simulink library "StateEstimation_lib"  (R2016b)
settings: Solver=VariableStepAuto  StartTime=0.0  StopTime=10.0  RelTol=1e-3
values from neighbouring files (symbols this model uses):
  accel_bias_init = zeros(3,1)    [Copy_of_StateEstimator_RIEKF.m]    (also in Quaternion_EKF.m; RightInvariant_EKF.m; StateEstimator_EKF.m; StateEstimator_RIEKF.m)
  accel_bias_noise_std = 0.1*ones(3,1)    [Copy_of_StateEstimator_RIEKF.m]    (also in Quaternion_EKF.m; RightInvariant_EKF.m; StateEstimator_EKF.m; StateEstimator_RIEKF.m)
  accel_noise_std = 0.1*ones(3,1)    [Copy_of_StateEstimator_RIEKF.m]    (also in Quaternion_EKF.m; RightInvariant_EKF.m; StateEstimator_EKF.m; StateEstimator_RIEKF.m)
  gyro_bias_init = zeros(3,1)    [Copy_of_StateEstimator_RIEKF.m]    (also in Quaternion_EKF.m; RightInvariant_EKF.m; StateEstimator_EKF.m; StateEstimator_RIEKF.m)
  gyro_bias_noise_std = 0.1*ones(3,1)    [Copy_of_StateEstimator_RIEKF.m]    (also in Quaternion_EKF.m; RightInvariant_EKF.m; StateEstimator_EKF.m; StateEstimator_RIEKF.m)
  gyro_noise_std = 0.1*ones(3,1)    [Copy_of_StateEstimator_RIEKF.m]    (also in Quaternion_EKF.m; RightInvariant_EKF.m; StateEstimator_EKF.m; StateEstimator_RIEKF.m)
undefined symbols (not defined in the file or in its folder): cassieParameters, CassieParameters, EKF_SampleTime, q_init, v_init
libraries: xpcutilitieslib x41, xpcrtudplib x41, dspfdesign x10, simulink x6, slrtlib x5
(part 1 of 4)
settings Model: Creator=Ross Hartley  LastModifiedBy=Ross Hartley

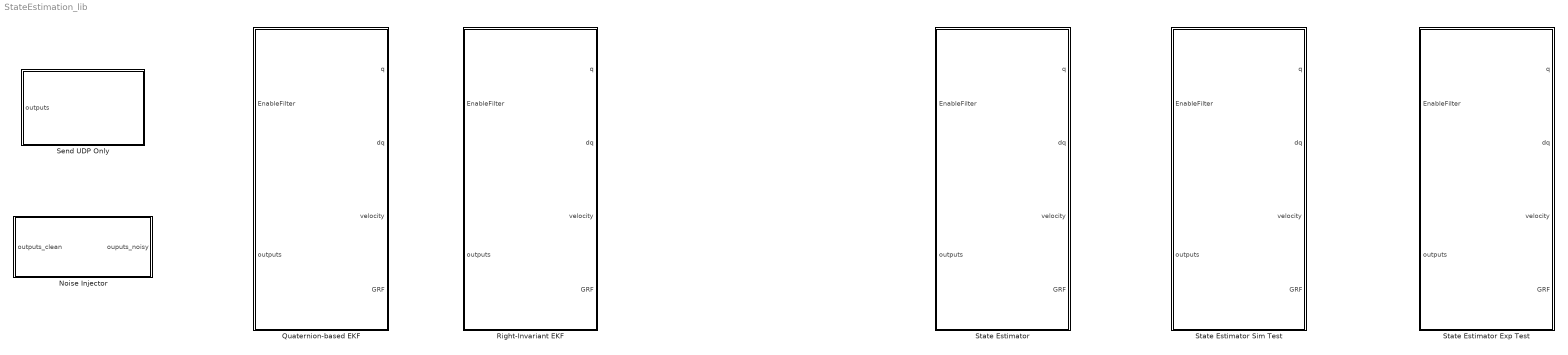
== system StateEstimation_lib ==
  Noise Injector : Subsystem
  Quaternion-based EKF : Subsystem
  Right-Invariant EKF : Subsystem
  Send UDP Only : Subsystem
  State Estimator : Subsystem
  State Estimator Exp Test : Subsystem
  State Estimator Sim Test : Subsystem

== system StateEstimation_lib/Noise Injector ==
  outputs_clean : Inport
  Bus Creator : BusCreator  Inputs=13  OutDataTypeStr=Bus: cassieOutputsBus
  Bus Selector1 : BusSelector  OutputSignals=vectorNavOrientation,vectorNavAngularVelocity,vectorNavLinearAcceleration,vectorNavMagneticField,vectorNavPressure,vectorNavTemperature,motorPosition,motorVelocity,jointPosition,jointVelocity,radio,stateOfCharge,status
  Inject Angular Velocity Noise : Subsystem
  Inject Linear Acceleration Noise : Subsystem
  ouputs_noisy : Outport
  wires:
  Inject Linear Acceleration Noise/1(a_noisy) -> Bus Creator/3  "vectorNavLinearAcceleration"
  Inject Angular Velocity Noise/1(w_noisy) -> Bus Creator/2  "vectorNavAngularVelocity"
  Bus Selector1/2 -> Inject Angular Velocity Noise/1(w_clean)  "<vectorNavAngularVelocity>"
  Bus Creator/1 -> ouputs_noisy/1
  outputs_clean/1 -> Bus Selector1/1
  Bus Selector1/11 -> Bus Creator/11  "<radio>"
  Bus Selector1/12 -> Bus Creator/12  "<stateOfCharge>"
  Bus Selector1/9 -> Bus Creator/9  "<jointPosition>"
  Bus Selector1/13 -> Bus Creator/13  "<status>"
  Bus Selector1/10 -> Bus Creator/10  "<jointVelocity>"
  Bus Selector1/8 -> Bus Creator/8  "<motorVelocity>"
  Bus Selector1/3 -> Inject Linear Acceleration Noise/1(a_clean)  "<vectorNavLinearAcceleration>"
  Bus Selector1/4 -> Bus Creator/4  "<vectorNavMagneticField>"
  Bus Selector1/7 -> Bus Creator/7  "<motorPosition>"
  Bus Selector1/5 -> Bus Creator/5  "<vectorNavPressure>"
  Bus Selector1/6 -> Bus Creator/6  "<vectorNavTemperature>"
  Bus Selector1/1 -> Bus Creator/1  "<vectorNavOrientation>"

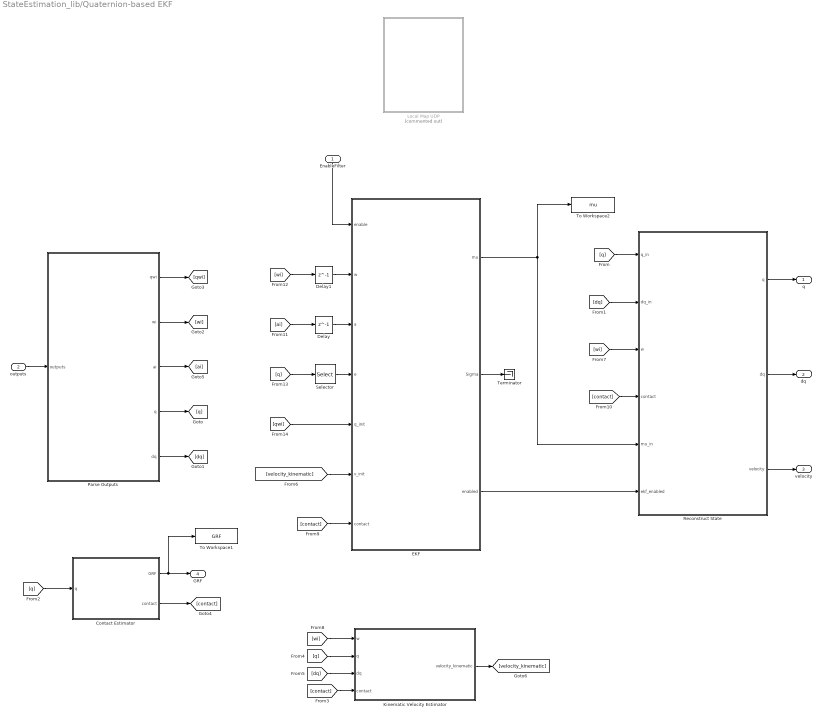
== system StateEstimation_lib/Quaternion-based EKF ==
  EnableFilter : Inport
  outputs : Inport  Port=2
  Contact Estimator : Subsystem
  Delay : Delay  DelayLength=1  InitialCondition=0
  Delay1 : Delay  DelayLength=1  InitialCondition=0
  EKF : Subsystem
  Kinematic Velocity Estimator : Subsystem
  Local Map UDP : Subsystem  Commented=on
  Parse Outputs : Subsystem
  Reconstruct State : Subsystem
  Selector : Selector  InputPortWidth=20  IndexOptions=Index vector (dialog)  Indices=[7:20]  OutputSizes=1
  Terminator : Terminator
  To Workspace1 : ToWorkspace  VariableName=GRF  SaveFormat=Timeseries  SampleTime=-1
  To Workspace2 : ToWorkspace  VariableName=mu  SaveFormat=Timeseries  SampleTime=-1
  q : Outport
  dq : Outport  Port=2
  velocity : Outport  Port=3
  GRF : Outport  Port=4
  wires:
  EKF/2(Sigma) -> Terminator/1
  EnableFilter/1 -> EKF/1(enable)
  [contact] -> EKF/7(contact)
  [ai] -> Delay/1
  [wi] -> Delay1/1
  [q] -> Selector/1
  outputs/1 -> Parse Outputs/1(outputs)
  Parse Outputs/3(ai) -> [ai]
  Parse Outputs/2(wi) -> [wi]
  Parse Outputs/4(q) -> [q]
  Parse Outputs/5(dq) -> [dq]
  Parse Outputs/1(qwi) -> [qwi]
  [q] -> Reconstruct State/1(q_in)
  [dq] -> Reconstruct State/2(dq_in)
  EKF/3(enabled) -> Reconstruct State/6(ekf_enabled)
  Reconstruct State/1(q) -> q/1
  Reconstruct State/2(dq) -> dq/1
  Reconstruct State/3(velocity) -> velocity/1
  Delay1/1 -> EKF/2(w)
  [wi] -> Reconstruct State/3(w)
  [contact] -> Reconstruct State/4(contact)
  [q] -> Contact Estimator/1(q)
  Contact Estimator/1(GRF) -> To Workspace1/1, GRF/1
  Contact Estimator/2(contact) -> [contact]
  EKF/1(mu) -> To Workspace2/1, Reconstruct State/5(mu_in)
  [wi] -> Kinematic Velocity Estimator/1(w)
  [q] -> Kinematic Velocity Estimator/2(q)
  [dq] -> Kinematic Velocity Estimator/3(dq)
  [contact] -> Kinematic Velocity Estimator/4(contact)
  Kinematic Velocity Estimator/1(velocity_kinematic) -> [velocity_kinematic]
  Delay/1 -> EKF/3(a)
  Selector/1 -> EKF/4(e)
  [qwi] -> EKF/5(q_init)
  [velocity_kinematic] -> EKF/6(v_init)

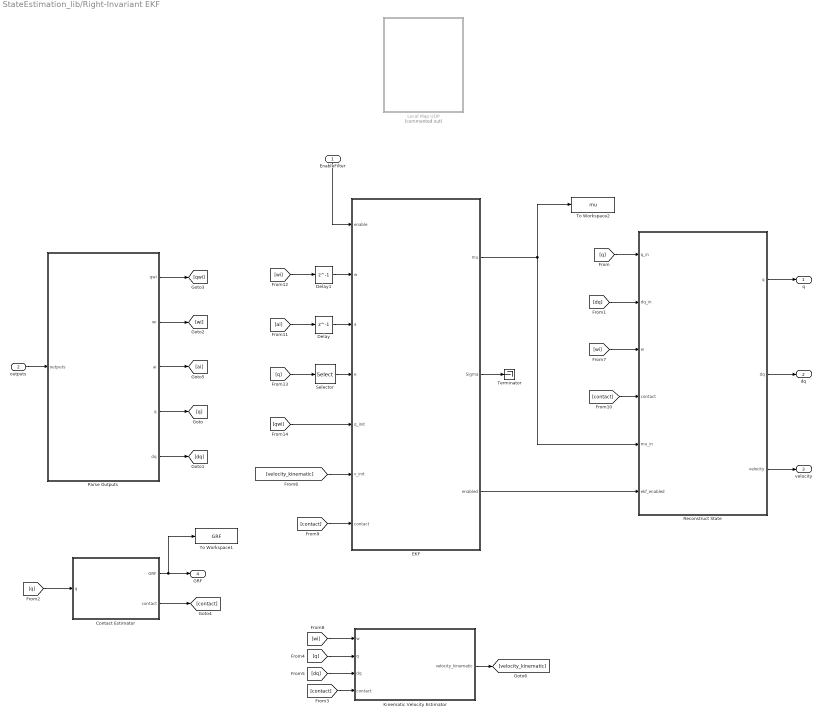
== system StateEstimation_lib/Right-Invariant EKF ==
  EnableFilter : Inport
  outputs : Inport  Port=2
  Contact Estimator : Subsystem
  Delay : Delay  DelayLength=1  InitialCondition=0
  Delay1 : Delay  DelayLength=1  InitialCondition=0
  EKF : Subsystem
  Kinematic Velocity Estimator : Subsystem
  Local Map UDP : Subsystem  Commented=on
  Parse Outputs : Subsystem
  Reconstruct State : Subsystem
  Selector : Selector  InputPortWidth=20  IndexOptions=Index vector (dialog)  Indices=[7:20]  OutputSizes=1
  Terminator : Terminator
  To Workspace1 : ToWorkspace  VariableName=GRF  SaveFormat=Timeseries  SampleTime=-1
  To Workspace2 : ToWorkspace  VariableName=mu  SaveFormat=Timeseries  SampleTime=-1
  q : Outport
  dq : Outport  Port=2
  velocity : Outport  Port=3
  GRF : Outport  Port=4
  wires:
  EKF/2(Sigma) -> Terminator/1
  EnableFilter/1 -> EKF/1(enable)
  [contact] -> EKF/7(contact)
  [ai] -> Delay/1
  [wi] -> Delay1/1
  [q] -> Selector/1
  outputs/1 -> Parse Outputs/1(outputs)
  Parse Outputs/3(ai) -> [ai]
  Parse Outputs/2(wi) -> [wi]
  Parse Outputs/4(q) -> [q]
  Parse Outputs/5(dq) -> [dq]
  Parse Outputs/1(qwi) -> [qwi]
  [q] -> Reconstruct State/1(q_in)
  [dq] -> Reconstruct State/2(dq_in)
  EKF/3(enabled) -> Reconstruct State/6(ekf_enabled)
  Reconstruct State/1(q) -> q/1
  Reconstruct State/2(dq) -> dq/1
  Reconstruct State/3(velocity) -> velocity/1
  Delay1/1 -> EKF/2(w)
  [wi] -> Reconstruct State/3(w)
  [contact] -> Reconstruct State/4(contact)
  [q] -> Contact Estimator/1(q)
  Contact Estimator/1(GRF) -> To Workspace1/1, GRF/1
  Contact Estimator/2(contact) -> [contact]
  EKF/1(mu) -> To Workspace2/1, Reconstruct State/5(mu_in)
  [wi] -> Kinematic Velocity Estimator/1(w)
  [q] -> Kinematic Velocity Estimator/2(q)
  [dq] -> Kinematic Velocity Estimator/3(dq)
  [contact] -> Kinematic Velocity Estimator/4(contact)
  Kinematic Velocity Estimator/1(velocity_kinematic) -> [velocity_kinematic]
  Delay/1 -> EKF/3(a)
  Selector/1 -> EKF/4(e)
  [qwi] -> EKF/5(q_init)
  [velocity_kinematic] -> EKF/6(v_init)

== system StateEstimation_lib/Send UDP Only ==
  outputs : Inport
  Constant : Constant  Value=[zeros(6,1), [0;0;0;1], zeros(12,1)]
  Constant1 : Constant  Value=eye(21,21)
  Constant2 : Constant  Value=0
  Contact Estimator : Subsystem
  Parse Outputs : Subsystem
  Send Pose UDP : Subsystem
  Terminator : Terminator
  wires:
  outputs/1 -> Parse Outputs/1(outputs)
  Parse Outputs/3(ai) -> [ai]
  Parse Outputs/2(wi) -> [wi]
  Parse Outputs/4(q) -> [q]
  Parse Outputs/5(dq) -> [dq]
  Parse Outputs/1(qwi) -> [qwi]
  [q] -> Contact Estimator/1(q)
  Contact Estimator/1(GRF) -> Terminator/1
  Contact Estimator/2(contact) -> [contact]
  Constant/1 -> Send Pose UDP/1(mu)
  Constant1/1 -> Send Pose UDP/2(Sigma)
  Constant2/1 -> Send Pose UDP/3(enabled)

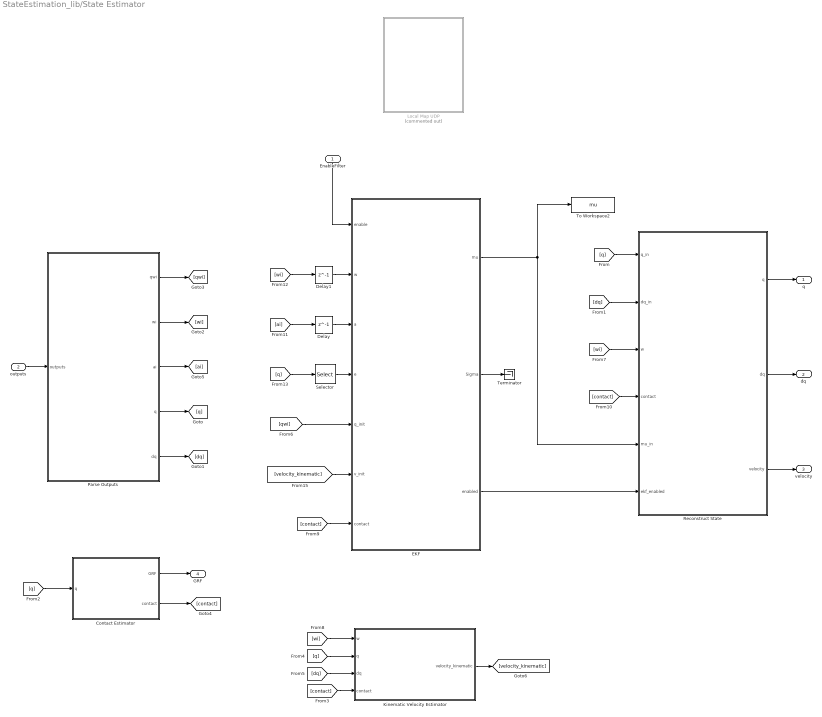
== system StateEstimation_lib/State Estimator ==
  EnableFilter : Inport
  outputs : Inport  Port=2
  Contact Estimator : Subsystem
  Delay : Delay  DelayLength=1  InitialCondition=0
  Delay1 : Delay  DelayLength=1  InitialCondition=0
  EKF : Subsystem
  Kinematic Velocity Estimator : Subsystem
  Local Map UDP : Subsystem  Commented=on
  Parse Outputs : Subsystem
  Reconstruct State : Subsystem
  Selector : Selector  InputPortWidth=20  IndexOptions=Index vector (dialog)  Indices=[7:20]  OutputSizes=1
  Terminator : Terminator
  To Workspace2 : ToWorkspace  VariableName=mu  SaveFormat=Timeseries  SampleTime=-1
  q : Outport
  dq : Outport  Port=2
  velocity : Outport  Port=3
  GRF : Outport  Port=4
  wires:
  EKF/2(Sigma) -> Terminator/1
  [velocity_kinematic] -> EKF/6(v_init)
  EnableFilter/1 -> EKF/1(enable)
  [contact] -> EKF/7(contact)
  [ai] -> Delay/1
  [wi] -> Delay1/1
  [q] -> Selector/1
  outputs/1 -> Parse Outputs/1(outputs)
  Parse Outputs/3(ai) -> [ai]
  Parse Outputs/2(wi) -> [wi]
  Parse Outputs/4(q) -> [q]
  Parse Outputs/5(dq) -> [dq]
  Parse Outputs/1(qwi) -> [qwi]
  [q] -> Reconstruct State/1(q_in)
  [dq] -> Reconstruct State/2(dq_in)
  EKF/3(enabled) -> Reconstruct State/6(ekf_enabled)
  Reconstruct State/1(q) -> q/1
  Reconstruct State/2(dq) -> dq/1
  Reconstruct State/3(velocity) -> velocity/1
  Delay1/1 -> EKF/2(w)
  [wi] -> Reconstruct State/3(w)
  [contact] -> Reconstruct State/4(contact)
  [q] -> Contact Estimator/1(q)
  Contact Estimator/1(GRF) -> GRF/1
  Contact Estimator/2(contact) -> [contact]
  EKF/1(mu) -> To Workspace2/1, Reconstruct State/5(mu_in)
  [wi] -> Kinematic Velocity Estimator/1(w)
  [q] -> Kinematic Velocity Estimator/2(q)
  [dq] -> Kinematic Velocity Estimator/3(dq)
  [contact] -> Kinematic Velocity Estimator/4(contact)
  Kinematic Velocity Estimator/1(velocity_kinematic) -> [velocity_kinematic]
  Delay/1 -> EKF/3(a)
  Selector/1 -> EKF/4(e)
  [qwi] -> EKF/5(q_init)

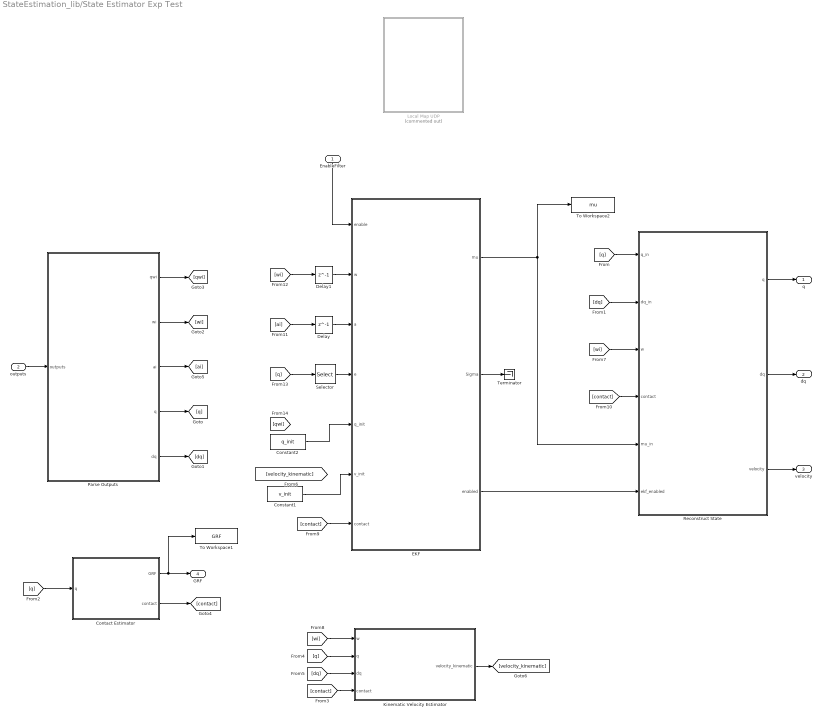
== system StateEstimation_lib/State Estimator Exp Test ==
  EnableFilter : Inport
  outputs : Inport  Port=2
  Constant1 : Constant  Value=v_init
  Constant2 : Constant  Value=q_init
  Contact Estimator : Subsystem
  Delay : Delay  DelayLength=1  InitialCondition=0
  Delay1 : Delay  DelayLength=1  InitialCondition=0
  EKF : Subsystem
  Kinematic Velocity Estimator : Subsystem
  Local Map UDP : Subsystem  Commented=on
  Parse Outputs : Subsystem
  Reconstruct State : Subsystem
  Selector : Selector  InputPortWidth=20  IndexOptions=Index vector (dialog)  Indices=[7:20]  OutputSizes=1
  Terminator : Terminator
  To Workspace1 : ToWorkspace  VariableName=GRF  SaveFormat=Timeseries  SampleTime=-1
  To Workspace2 : ToWorkspace  VariableName=mu  SaveFormat=Timeseries  SampleTime=-1
  q : Outport
  dq : Outport  Port=2
  velocity : Outport  Port=3
  GRF : Outport  Port=4
  wires:
  EKF/2(Sigma) -> Terminator/1
  EnableFilter/1 -> EKF/1(enable)
  [contact] -> EKF/7(contact)
  [ai] -> Delay/1
  [wi] -> Delay1/1
  [q] -> Selector/1
  outputs/1 -> Parse Outputs/1(outputs)
  Parse Outputs/3(ai) -> [ai]
  Parse Outputs/2(wi) -> [wi]
  Parse Outputs/4(q) -> [q]
  Parse Outputs/5(dq) -> [dq]
  Parse Outputs/1(qwi) -> [qwi]
  [q] -> Reconstruct State/1(q_in)
  [dq] -> Reconstruct State/2(dq_in)
  EKF/3(enabled) -> Reconstruct State/6(ekf_enabled)
  Reconstruct State/1(q) -> q/1
  Reconstruct State/2(dq) -> dq/1
  Reconstruct State/3(velocity) -> velocity/1
  Delay1/1 -> EKF/2(w)
  [wi] -> Reconstruct State/3(w)
  [contact] -> Reconstruct State/4(contact)
  [q] -> Contact Estimator/1(q)
  Contact Estimator/1(GRF) -> To Workspace1/1, GRF/1
  Contact Estimator/2(contact) -> [contact]
  EKF/1(mu) -> To Workspace2/1, Reconstruct State/5(mu_in)
  [wi] -> Kinematic Velocity Estimator/1(w)
  [q] -> Kinematic Velocity Estimator/2(q)
  [dq] -> Kinematic Velocity Estimator/3(dq)
  [contact] -> Kinematic Velocity Estimator/4(contact)
  Kinematic Velocity Estimator/1(velocity_kinematic) -> [velocity_kinematic]
  Delay/1 -> EKF/3(a)
  Selector/1 -> EKF/4(e)
  Constant2/1 -> EKF/5(q_init)
  Constant1/1 -> EKF/6(v_init)

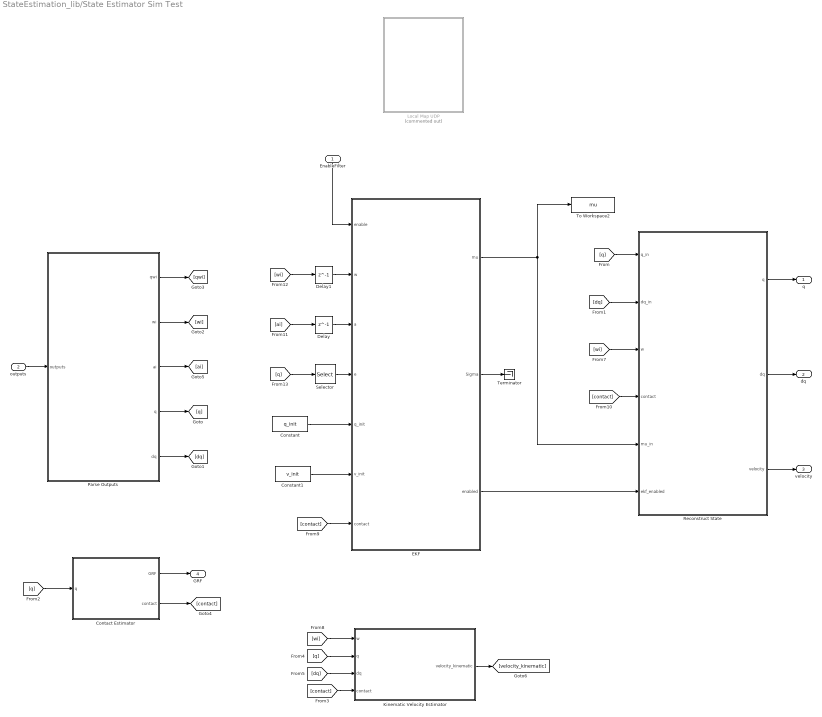
== system StateEstimation_lib/State Estimator Sim Test ==
  EnableFilter : Inport
  outputs : Inport  Port=2
  Constant : Constant  Value=q_init
  Constant1 : Constant  Value=v_init
  Contact Estimator : Subsystem
  Delay : Delay  DelayLength=1  InitialCondition=0
  Delay1 : Delay  DelayLength=1  InitialCondition=0
  EKF : Subsystem
  Kinematic Velocity Estimator : Subsystem
  Local Map UDP : Subsystem  Commented=on
  Parse Outputs : Subsystem
  Reconstruct State : Subsystem
  Selector : Selector  InputPortWidth=20  IndexOptions=Index vector (dialog)  Indices=[7:20]  OutputSizes=1
  Terminator : Terminator
  To Workspace2 : ToWorkspace  VariableName=mu  SaveFormat=Timeseries  SampleTime=-1
  q : Outport
  dq : Outport  Port=2
  velocity : Outport  Port=3
  GRF : Outport  Port=4
  wires:
  EKF/2(Sigma) -> Terminator/1
  EnableFilter/1 -> EKF/1(enable)
  [contact] -> EKF/7(contact)
  [ai] -> Delay/1
  [wi] -> Delay1/1
  [q] -> Selector/1
  outputs/1 -> Parse Outputs/1(outputs)
  Parse Outputs/3(ai) -> [ai]
  Parse Outputs/2(wi) -> [wi]
  Parse Outputs/4(q) -> [q]
  Parse Outputs/5(dq) -> [dq]
  Parse Outputs/1(qwi) -> [qwi]
  [q] -> Reconstruct State/1(q_in)
  [dq] -> Reconstruct State/2(dq_in)
  EKF/3(enabled) -> Reconstruct State/6(ekf_enabled)
  Reconstruct State/1(q) -> q/1
  Reconstruct State/2(dq) -> dq/1
  Reconstruct State/3(velocity) -> velocity/1
  Delay1/1 -> EKF/2(w)
  [wi] -> Reconstruct State/3(w)
  [contact] -> Reconstruct State/4(contact)
  [q] -> Contact Estimator/1(q)
  Contact Estimator/1(GRF) -> GRF/1
  Contact Estimator/2(contact) -> [contact]
  EKF/1(mu) -> To Workspace2/1, Reconstruct State/5(mu_in)
  [wi] -> Kinematic Velocity Estimator/1(w)
  [q] -> Kinematic Velocity Estimator/2(q)
  [dq] -> Kinematic Velocity Estimator/3(dq)
  [contact] -> Kinematic Velocity Estimator/4(contact)
  Kinematic Velocity Estimator/1(velocity_kinematic) -> [velocity_kinematic]
  Delay/1 -> EKF/3(a)
  Selector/1 -> EKF/4(e)
  Constant1/1 -> EKF/6(v_init)
  Constant/1 -> EKF/5(q_init)

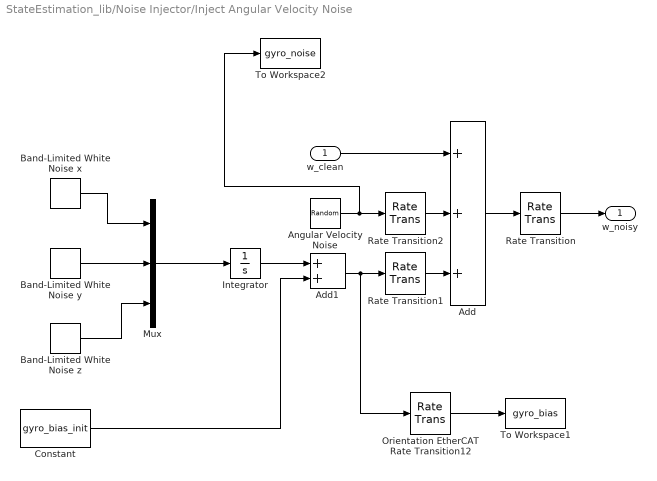
== system StateEstimation_lib/Noise Injector/Inject Angular Velocity Noise ==
  w_clean : Inport
  Add : Sum  Inputs=+++
  Add1 : Sum
  Angular Velocity Noise : RandomNumber  Mean=[0;0;0]  Variance=[gyro_noise_std(1)^2; gyro_noise_std(2)^2; gyro_noise_std(3)^2]  Seed=[7;8;9]  SampleTime=cassieParameters.vectorNavSampleTime
  Band-Limited White Noise x : simulink/Sources/Band-Limited White Noise  Cov=[gyro_bias_noise_std(1)^2]  Ts=cassieParameters.etherCatSampleTime  seed=[1]
  Band-Limited White Noise y : simulink/Sources/Band-Limited White Noise  Cov=[gyro_bias_noise_std(2)^2]  Ts=cassieParameters.etherCatSampleTime  seed=[2]
  Band-Limited White Noise z : simulink/Sources/Band-Limited White Noise  Cov=[gyro_bias_noise_std(3)^2]  Ts=cassieParameters.etherCatSampleTime  seed=[3]
  Constant : Constant  Value=gyro_bias_init
  Integrator : Integrator  InitialCondition=[0;0;0]
  Mux : Mux  Inputs=3
  Orientation EtherCAT Rate Transition12 : RateTransition  Deterministic=off  OutPortSampleTime=CassieParameters.etherCatSampleTime
  Rate Transition : RateTransition  OutPortSampleTime=cassieParameters.etherCatSampleTime
  Rate Transition1 : RateTransition  Deterministic=off  OutPortSampleTime=cassieParameters.etherCatSampleTime
  Rate Transition2 : RateTransition  Deterministic=off  OutPortSampleTime=cassieParameters.etherCatSampleTime
  To Workspace1 : ToWorkspace  VariableName=gyro_bias  SaveFormat=Timeseries  SampleTime=-1
  To Workspace2 : ToWorkspace  VariableName=gyro_noise  SaveFormat=Timeseries  SampleTime=-1
  w_noisy : Outport
  wires:
  Add/1 -> Rate Transition/1
  Rate Transition/1 -> w_noisy/1
  Mux/1 -> Integrator/1
  Band-Limited White Noise z/1 -> Mux/3
  Band-Limited White Noise y/1 -> Mux/2
  Band-Limited White Noise x/1 -> Mux/1
  Integrator/1 -> Add1/1
  Angular Velocity Noise/1 -> To Workspace2/1, Rate Transition2/1
  w_clean/1 -> Add/1
  Add1/1 -> Orientation EtherCAT Rate Transition12/1, Rate Transition1/1
  Constant/1 -> Add1/2
  Rate Transition1/1 -> Add/3
  Rate Transition2/1 -> Add/2
  Orientation EtherCAT Rate Transition12/1 -> To Workspace1/1

== system StateEstimation_lib/Noise Injector/Inject Linear Acceleration Noise ==
  a_clean : Inport
  Add : Sum  Inputs=+++
  Add1 : Sum
  Band-Limited White Noise x : simulink/Sources/Band-Limited White Noise  Cov=[accel_bias_noise_std(1)^2]  Ts=cassieParameters.etherCatSampleTime  seed=[4]
  Band-Limited White Noise y : simulink/Sources/Band-Limited White Noise  Cov=[accel_bias_noise_std(2)^2]  Ts=cassieParameters.etherCatSampleTime  seed=[5]
  Band-Limited White Noise z : simulink/Sources/Band-Limited White Noise  Cov=[accel_bias_noise_std(3)^2]  Ts=cassieParameters.etherCatSampleTime  seed=[6]
  Initial Bias : Constant  Value=accel_bias_init
  Integrator : Integrator  InitialCondition=[0;0;0]
  Linear Acceleration Noise : RandomNumber  Mean=[0;0;0]  Variance=[accel_noise_std(1)^2; accel_noise_std(2)^2; accel_noise_std(3)^2]  Seed=[10;11;12]  SampleTime=cassieParameters.vectorNavSampleTime
  Mux : Mux  Inputs=3
  Orientation EtherCAT Rate Transition12 : RateTransition  Deterministic=off  OutPortSampleTime=CassieParameters.etherCatSampleTime
  Rate Transition1 : RateTransition  Deterministic=off  OutPortSampleTime=cassieParameters.etherCatSampleTime
  Rate Transition2 : RateTransition  Deterministic=off  OutPortSampleTime=cassieParameters.etherCatSampleTime
  To Workspace1 : ToWorkspace  VariableName=accel_bias  SaveFormat=Timeseries  SampleTime=-1
  To Workspace2 : ToWorkspace  VariableName=accel_noise  SaveFormat=Timeseries  SampleTime=-1
  a_noisy : Outport
  wires:
  Add/1 -> a_noisy/1
  Integrator/1 -> Add1/1
  Mux/1 -> Integrator/1
  Band-Limited White Noise z/1 -> Mux/3
  Band-Limited White Noise y/1 -> Mux/2
  Band-Limited White Noise x/1 -> Mux/1
  Linear Acceleration Noise/1 -> To Workspace2/1, Rate Transition1/1
  a_clean/1 -> Add/1
  Initial Bias/1 -> Add1/2
  Add1/1 -> Orientation EtherCAT Rate Transition12/1, Rate Transition2/1
  Rate Transition1/1 -> Add/2
  Rate Transition2/1 -> Add/3
  Orientation EtherCAT Rate Transition12/1 -> To Workspace1/1

== system StateEstimation_lib/Quaternion-based EKF/Contact Estimator ==
  q : Inport
  GRF_Estimator : MATLAB Function  TreatAsAtomicUnit=on
  Selector : Selector  InputPortWidth=4  IndexOptions=Index vector (dialog)  Indices=[2, 4]  OutputSizes=1
  Send Contact : Subsystem
  GRF : Outport
  contact : Outport  Port=2
  wires:
  GRF_Estimator/1(GRF) -> Selector/1, GRF/1
  GRF_Estimator/2(contact) -> contact/1
  q/1 -> GRF_Estimator/1(q)
  Selector/1 -> Send Contact/1(contact)

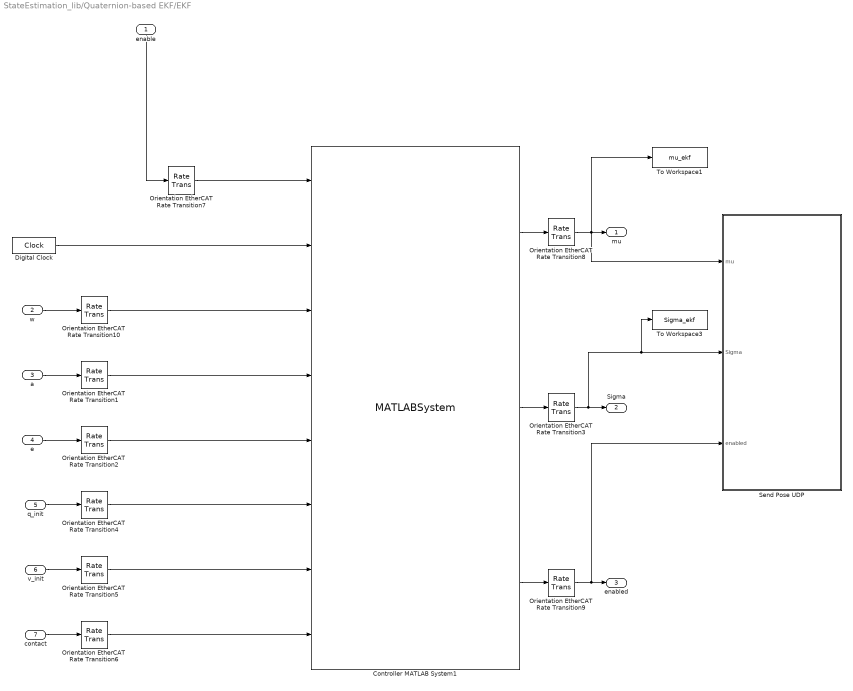
== system StateEstimation_lib/Quaternion-based EKF/EKF ==
  enable : Inport
  w : Inport  Port=2
  a : Inport  Port=3
  e : Inport  Port=4
  q_init : Inport  Port=5
  v_init : Inport  Port=6
  contact : Inport  Port=7
  Controller MATLAB System1 : MATLABSystem  System=StateEstimator_EKF  static_bias_initialization=static_bias_initialization  ekf_update_enabled=true  dt=EKF_SampleTime  enable_bias_estimation=enable_bias_estimation  gyro_noise_std=gyro_noise_std  gyro_bias_noise_std=gyro_bias_noise_std  accel_noise_std=accel_noise_std  accel_bias_noise_std=accel_bias_noise_std  contact_noise_std=contact_noise_std  encoder_noise_std=encoder_noise_std  gyro_bias_init=gyro_bias_init  accel_bias_init=accel_bias_init  SimulateUsing=Code generation
      mask Type: StateEstimator_EKF
      mask Display:
      | disp('StateEstimator_EKF');
      | port_label('input',1,'EnableFilter');
      | port_label('input',2,'t');
      | port_label('input',3,'w');
      | port_label('input',4,'a');
      | port_label('input',5,'e');
      | port_label('input',6,'q_init');
      | port_label('input',7,'v_init');
      | port_label('input',8,'contact');
      | port_label('output',1,'mu');
      | port_label('output',2,'Sigma');
      | port_label('output',3,'enabled');
  Digital Clock : DigitalClock  SampleTime=EKF_SampleTime
  Orientation EtherCAT Rate Transition{1..2,4..7,10} (7 alike) : RateTransition  Deterministic=off  OutPortSampleTime=EKF_SampleTime
  Orientation EtherCAT Rate Transition3 : RateTransition  Deterministic=off  OutPortSampleTime=CassieParameters.etherCatSampleTime
  Orientation EtherCAT Rate Transition8 : RateTransition  Deterministic=off  OutPortSampleTime=CassieParameters.etherCatSampleTime
  Orientation EtherCAT Rate Transition9 : RateTransition  Deterministic=off  OutPortSampleTime=CassieParameters.etherCatSampleTime
  Send Pose UDP : Subsystem
  To Workspace1 : ToWorkspace  VariableName=mu_ekf  SaveFormat=Timeseries  SampleTime=-1
  To Workspace3 : ToWorkspace  VariableName=Sigma_ekf  SaveFormat=Timeseries  SampleTime=-1
  mu : Outport
  Sigma : Outport  Port=2
  enabled : Outport  Port=3
  wires:
  enable/1 -> Orientation EtherCAT Rate Transition7/1
  Orientation EtherCAT Rate Transition7/1 -> Controller MATLAB System1/1
  Orientation EtherCAT Rate Transition8/1 -> To Workspace1/1, Send Pose UDP/1(mu), mu/1
  Digital Clock/1 -> Controller MATLAB System1/2
  Orientation EtherCAT Rate Transition9/1 -> Send Pose UDP/3(enabled), enabled/1
  Controller MATLAB System1/1 -> Orientation EtherCAT Rate Transition8/1
  Controller MATLAB System1/3 -> Orientation EtherCAT Rate Transition9/1
  Orientation EtherCAT Rate Transition6/1 -> Controller MATLAB System1/8
  Orientation EtherCAT Rate Transition5/1 -> Controller MATLAB System1/7
  q_init/1 -> Orientation EtherCAT Rate Transition4/1
  v_init/1 -> Orientation EtherCAT Rate Transition5/1
  contact/1 -> Orientation EtherCAT Rate Transition6/1
  w/1 -> Orientation EtherCAT Rate Transition10/1
  Orientation EtherCAT Rate Transition10/1 -> Controller MATLAB System1/3
  a/1 -> Orientation EtherCAT Rate Transition1/1
  e/1 -> Orientation EtherCAT Rate Transition2/1
  Controller MATLAB System1/2 -> Orientation EtherCAT Rate Transition3/1
  Orientation EtherCAT Rate Transition3/1 -> To Workspace3/1, Send Pose UDP/2(Sigma), Sigma/1
  Orientation EtherCAT Rate Transition1/1 -> Controller MATLAB System1/4
  Orientation EtherCAT Rate Transition2/1 -> Controller MATLAB System1/5
  Orientation EtherCAT Rate Transition4/1 -> Controller MATLAB System1/6

== system StateEstimation_lib/Quaternion-based EKF/Kinematic Velocity Estimator ==
  w : Inport
  q : Inport  Port=2
  dq : Inport  Port=3
  contact : Inport  Port=4
  Kinematic_Velocity : MATLAB Function  TreatAsAtomicUnit=on
  Selector2 : Selector  InputPortWidth=20  IndexOptions=Index vector (dialog)  Indices=[7:20]  OutputSizes=1
  Selector3 : Selector  InputPortWidth=20  IndexOptions=Index vector (dialog)  Indices=[7:20]  OutputSizes=1
  velocity_kinematic : Outport
  wires:
  w/1 -> Kinematic_Velocity/1(w)
  contact/1 -> Kinematic_Velocity/4(contact)
  dq/1 -> Selector3/1
  Kinematic_Velocity/1(velocity) -> velocity_kinematic/1
  q/1 -> Selector2/1
  Selector3/1 -> Kinematic_Velocity/3(e_dot)
  Selector2/1 -> Kinematic_Velocity/2(e)

== system StateEstimation_lib/Quaternion-based EKF/Local Map UDP ==
  note: Local Map UDP Data Structure
      |
      | Map Information
      | double time
      | double resolution
      | double length_x
      | double length_y
      |
      | Map Center Pose
      | double position_x
      | double position_y
      | double position_z
      | double orientation_x
      | double orientation_y
      | double orientation_z
      | double orientation_w
      |
      | Update Block Data
      | double row_start_index
      | double column_start_index
      | double[100] elevation_data
  "Byte Unpacking " : xpcutilitieslib/Byte Unpacking   MaskUnpackedDataTypes={'double'}  MaskUnpackedDataSizes={[45]}  MaskAlignment=1
  Data Store Memory : DataStoreMemory  DataStoreName=local_map  ReadBeforeWriteMsg=warning  WriteAfterWriteMsg=warning  WriteAfterReadMsg=warning  ShowAdditionalParam=off
  Data Store Write : DataStoreWrite  DataStoreName=local_map
  Receive : xpcrtudplib/UDP Receive  ipAddressVal=Use host-target connection  localPort=25000  rcvWidth=45*8  rcvFmAny=off  fmAddress=10.10.10.5  sampleTime=-1
  Terminator : Terminator
  wires:
  Receive/2 -> Terminator/1
  Receive/1 -> "Byte Unpacking "/1
  "Byte Unpacking "/1 -> Data Store Write/1

== system StateEstimation_lib/Quaternion-based EKF/Parse Outputs ==
  outputs : Inport
  Bus Selector : BusSelector  OutputSignals=radio
  Parse_Outputs : MATLAB Function  TreatAsAtomicUnit=on
  Send IMU UDP : Subsystem
  Send JointState UDP : Subsystem
  Send Radio : Subsystem
  Send Time : Subsystem
  qwi : Outport
  wi : Outport  Port=2
  ai : Outport  Port=3
  q : Outport  Port=4
  dq : Outport  Port=5
  wires:
  Bus Selector/1 -> Send Radio/1(radio)  "<radio>"
  Parse_Outputs/5(dq) -> dq/1, Send JointState UDP/2(dq)
  outputs/1 -> Bus Selector/1, Parse_Outputs/1(outputs)
  Parse_Outputs/2(wi) -> Send IMU UDP/2(w), wi/1
  Parse_Outputs/4(q) -> q/1, Send JointState UDP/1(q)
  Parse_Outputs/1(qwi) -> qwi/1, Send IMU UDP/1(q)
  Parse_Outputs/3(ai) -> Send IMU UDP/3(a), ai/1

== system StateEstimation_lib/Quaternion-based EKF/Reconstruct State ==
  q_in : Inport
  dq_in : Inport  Port=2
  w : Inport  Port=3
  contact : Inport  Port=4
  mu_in : Inport  Port=5
  ekf_enabled : Inport  Port=6
  Construct_State : MATLAB Function  TreatAsAtomicUnit=on
  Low Pass Filter : Subsystem  TreatAsAtomicUnit=on
  Mux : Mux
  Scope 6 : slrtlib/Displays and Logging/Scope   scopeno=2  scopetype=File  autostart=on  viewmode=Numerical  formatstr='%15.6f'  grid=on  ylimits=[0,0]  nosamples=250  noprepostsamples=0  interleave=1  triggermode=FreeRun  triggersignal=1  trigsignalfromport=on  triggerlevel=0.5  triggerslope=Rising  triggerscope=1  triggersample=0  filename=ekf1.dat  mode=Commit  writesize=512  autorestart=on  dynamicfilemode=off  maxwritefilesize=4000*1024^2
  q : Outport
  dq : Outport  Port=2
  velocity : Outport  Port=3
  wires:
  Low Pass Filter/1(filtered_signal) -> velocity/1
  mu_in/1 -> Construct_State/5(mu), Mux/3
  dq_in/1 -> Construct_State/2("dq ")
  Construct_State/1(q) -> q/1
  Construct_State/3(velocity) -> Mux/1, Low Pass Filter/1(signal)
  Construct_State/5(filter_selector) -> Low Pass Filter/2(selector)
  Mux/1 -> Scope 6/1
  q_in/1 -> Construct_State/1("q ")
  ekf_enabled/1 -> Construct_State/6(ekf_enabled), Mux/4
  Construct_State/2(dq) -> dq/1
  w/1 -> Construct_State/3(w)
  contact/1 -> Construct_State/4(contact)
  Construct_State/4(velocity_kinematic) -> Mux/2

== system StateEstimation_lib/Right-Invariant EKF/Contact Estimator ==
  q : Inport
  GRF_Estimator : MATLAB Function  TreatAsAtomicUnit=on
  Selector : Selector  InputPortWidth=4  IndexOptions=Index vector (dialog)  Indices=[2, 4]  OutputSizes=1
  Send Contact : Subsystem
  GRF : Outport
  contact : Outport  Port=2
  wires:
  GRF_Estimator/1(GRF) -> Selector/1, GRF/1
  GRF_Estimator/2(contact) -> contact/1
  q/1 -> GRF_Estimator/1(q)
  Selector/1 -> Send Contact/1(contact)

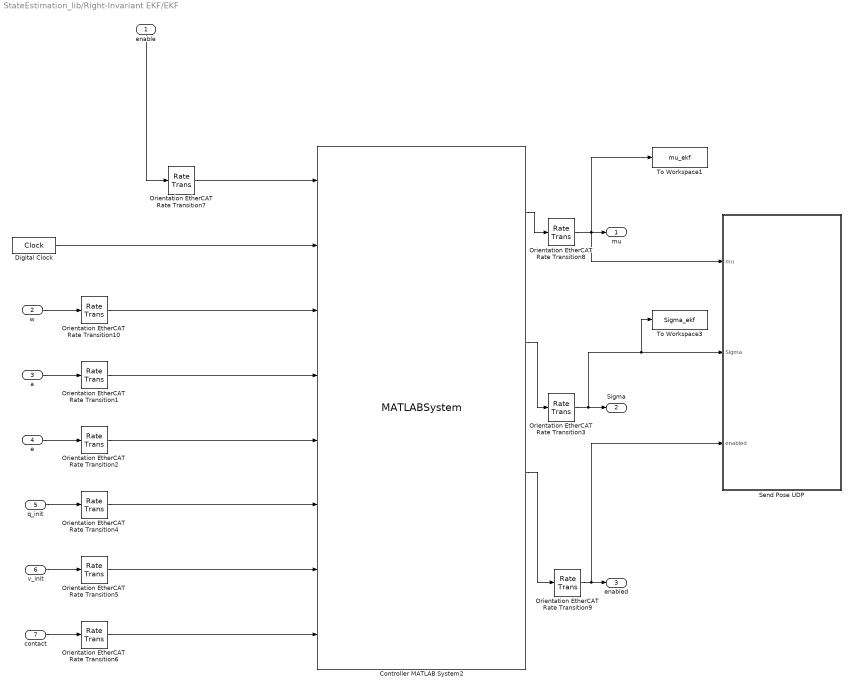
== system StateEstimation_lib/Right-Invariant EKF/EKF ==
  enable : Inport
  w : Inport  Port=2
  a : Inport  Port=3
  e : Inport  Port=4
  q_init : Inport  Port=5
  v_init : Inport  Port=6
  contact : Inport  Port=7
  Controller MATLAB System2 : MATLABSystem  System=StateEstimator_RIEKF  static_bias_initialization=static_bias_initialization  ekf_update_enabled=true  dt=EKF_SampleTime  enable_bias_estimation=enable_bias_estimation  gyro_noise_std=gyro_noise_std  gyro_bias_noise_std=gyro_bias_noise_std  accel_noise_std=accel_noise_std  accel_bias_noise_std=accel_bias_noise_std  contact_noise_std=contact_noise_std  encoder_noise_std=encoder_noise_std  gyro_bias_init=gyro_bias_init  accel_bias_init=accel_bias_init  SimulateUsing=Code generation
      mask Type: StateEstimator_RIEKF
      mask Display:
      | disp('StateEstimator_RIEKF');
      | port_label('input',1,'EnableFilter');
      | port_label('input',2,'t');
      | port_label('input',3,'w');
      | port_label('input',4,'a');
      | port_label('input',5,'e');
      | port_label('input',6,'q_init');
      | port_label('input',7,'v_init');
      | port_label('input',8,'contact');
      | port_label('output',1,'mu');
      | port_label('output',2,'Sigma');
      | port_label('output',3,'enabled');
      | port_label('output',4,'K');
  Digital Clock : DigitalClock  SampleTime=EKF_SampleTime
  Orientation EtherCAT Rate Transition{1..2,4..7,10} (7 alike) : RateTransition  Deterministic=off  OutPortSampleTime=EKF_SampleTime
  Orientation EtherCAT Rate Transition3 : RateTransition  Deterministic=off  OutPortSampleTime=CassieParameters.etherCatSampleTime
  Orientation EtherCAT Rate Transition8 : RateTransition  Deterministic=off  OutPortSampleTime=CassieParameters.etherCatSampleTime
  Orientation EtherCAT Rate Transition9 : RateTransition  Deterministic=off  OutPortSampleTime=CassieParameters.etherCatSampleTime
  Send Pose UDP : Subsystem
  To Workspace1 : ToWorkspace  VariableName=mu_ekf  SaveFormat=Timeseries  SampleTime=-1
  To Workspace3 : ToWorkspace  VariableName=Sigma_ekf  SaveFormat=Timeseries  SampleTime=-1
  mu : Outport
  Sigma : Outport  Port=2
  enabled : Outport  Port=3
  wires:
  enable/1 -> Orientation EtherCAT Rate Transition7/1
  Orientation EtherCAT Rate Transition7/1 -> Controller MATLAB System2/1
  Orientation EtherCAT Rate Transition8/1 -> To Workspace1/1, Send Pose UDP/1(mu), mu/1
  Digital Clock/1 -> Controller MATLAB System2/2
  Orientation EtherCAT Rate Transition9/1 -> Send Pose UDP/3(enabled), enabled/1
  Controller MATLAB System2/1 -> Orientation EtherCAT Rate Transition8/1
  Controller MATLAB System2/3 -> Orientation EtherCAT Rate Transition9/1
  Orientation EtherCAT Rate Transition6/1 -> Controller MATLAB System2/8
  Orientation EtherCAT Rate Transition5/1 -> Controller MATLAB System2/7
  q_init/1 -> Orientation EtherCAT Rate Transition4/1
  v_init/1 -> Orientation EtherCAT Rate Transition5/1
  contact/1 -> Orientation EtherCAT Rate Transition6/1
  w/1 -> Orientation EtherCAT Rate Transition10/1
  Orientation EtherCAT Rate Transition10/1 -> Controller MATLAB System2/3
  a/1 -> Orientation EtherCAT Rate Transition1/1
  e/1 -> Orientation EtherCAT Rate Transition2/1
  Controller MATLAB System2/2 -> Orientation EtherCAT Rate Transition3/1
  Orientation EtherCAT Rate Transition3/1 -> To Workspace3/1, Send Pose UDP/2(Sigma), Sigma/1
  Orientation EtherCAT Rate Transition1/1 -> Controller MATLAB System2/4
  Orientation EtherCAT Rate Transition2/1 -> Controller MATLAB System2/5
  Orientation EtherCAT Rate Transition4/1 -> Controller MATLAB System2/6

== system StateEstimation_lib/Right-Invariant EKF/Kinematic Velocity Estimator ==
  w : Inport
  q : Inport  Port=2
  dq : Inport  Port=3
  contact : Inport  Port=4
  Kinematic_Velocity : MATLAB Function  TreatAsAtomicUnit=on
  Selector2 : Selector  InputPortWidth=20  IndexOptions=Index vector (dialog)  Indices=[7:20]  OutputSizes=1
  Selector3 : Selector  InputPortWidth=20  IndexOptions=Index vector (dialog)  Indices=[7:20]  OutputSizes=1
  velocity_kinematic : Outport
  wires:
  w/1 -> Kinematic_Velocity/1(w)
  contact/1 -> Kinematic_Velocity/4(contact)
  dq/1 -> Selector3/1
  Kinematic_Velocity/1(velocity) -> velocity_kinematic/1
  q/1 -> Selector2/1
  Selector3/1 -> Kinematic_Velocity/3(e_dot)
  Selector2/1 -> Kinematic_Velocity/2(e)

== system StateEstimation_lib/Right-Invariant EKF/Local Map UDP ==
  note: Local Map UDP Data Structure
      |
      | Map Information
      | double time
      | double resolution
      | double length_x
      | double length_y
      |
      | Map Center Pose
      | double position_x
      | double position_y
      | double position_z
      | double orientation_x
      | double orientation_y
      | double orientation_z
      | double orientation_w
      |
      | Update Block Data
      | double row_start_index
      | double column_start_index
      | double[100] elevation_data
  "Byte Unpacking " : xpcutilitieslib/Byte Unpacking   MaskUnpackedDataTypes={'double'}  MaskUnpackedDataSizes={[45]}  MaskAlignment=1
  Data Store Memory : DataStoreMemory  DataStoreName=local_map  ReadBeforeWriteMsg=warning  WriteAfterWriteMsg=warning  WriteAfterReadMsg=warning  ShowAdditionalParam=off
  Data Store Write : DataStoreWrite  DataStoreName=local_map
  Receive : xpcrtudplib/UDP Receive  ipAddressVal=Use host-target connection  localPort=25000  rcvWidth=45*8  rcvFmAny=off  fmAddress=10.10.10.5  sampleTime=-1
  Terminator : Terminator
  wires:
  Receive/2 -> Terminator/1
  Receive/1 -> "Byte Unpacking "/1
  "Byte Unpacking "/1 -> Data Store Write/1

== system StateEstimation_lib/Right-Invariant EKF/Parse Outputs ==
  outputs : Inport
  Bus Selector : BusSelector  OutputSignals=radio
  Parse_Outputs : MATLAB Function  TreatAsAtomicUnit=on
  Send IMU UDP : Subsystem
  Send JointState UDP : Subsystem
  Send Radio : Subsystem
  Send Time : Subsystem
  qwi : Outport
  wi : Outport  Port=2
  ai : Outport  Port=3
  q : Outport  Port=4
  dq : Outport  Port=5
  wires:
  Bus Selector/1 -> Send Radio/1(radio)  "<radio>"
  Parse_Outputs/5(dq) -> dq/1, Send JointState UDP/2(dq)
  outputs/1 -> Bus Selector/1, Parse_Outputs/1(outputs)
  Parse_Outputs/2(wi) -> Send IMU UDP/2(w), wi/1
  Parse_Outputs/4(q) -> q/1, Send JointState UDP/1(q)
  Parse_Outputs/1(qwi) -> qwi/1, Send IMU UDP/1(q)
  Parse_Outputs/3(ai) -> Send IMU UDP/3(a), ai/1

== system StateEstimation_lib/Right-Invariant EKF/Reconstruct State ==
  q_in : Inport
  dq_in : Inport  Port=2
  w : Inport  Port=3
  contact : Inport  Port=4
  mu_in : Inport  Port=5
  ekf_enabled : Inport  Port=6
  Construct_State : MATLAB Function  TreatAsAtomicUnit=on
  Low Pass Filter : Subsystem  TreatAsAtomicUnit=on
  Mux : Mux
  Scope 6 : slrtlib/Displays and Logging/Scope   scopeno=2  scopetype=File  autostart=on  viewmode=Numerical  formatstr='%15.6f'  grid=on  ylimits=[0,0]  nosamples=250  noprepostsamples=0  interleave=1  triggermode=FreeRun  triggersignal=1  trigsignalfromport=on  triggerlevel=0.5  triggerslope=Rising  triggerscope=1  triggersample=0  filename=ekf1.dat  mode=Commit  writesize=512  autorestart=on  dynamicfilemode=off  maxwritefilesize=4000*1024^2
  q : Outport
  dq : Outport  Port=2
  velocity : Outport  Port=3
  wires:
  Low Pass Filter/1(filtered_signal) -> velocity/1
  mu_in/1 -> Construct_State/5(mu), Mux/3
  dq_in/1 -> Construct_State/2("dq ")
  Construct_State/1(q) -> q/1
  Construct_State/3(velocity) -> Mux/1, Low Pass Filter/1(signal)
  Construct_State/5(filter_selector) -> Low Pass Filter/2(selector)
  Mux/1 -> Scope 6/1
  q_in/1 -> Construct_State/1("q ")
  ekf_enabled/1 -> Construct_State/6(ekf_enabled), Mux/4
  Construct_State/2(dq) -> dq/1
  w/1 -> Construct_State/3(w)
  contact/1 -> Construct_State/4(contact)
  Construct_State/4(velocity_kinematic) -> Mux/2

== system StateEstimation_lib/Send UDP Only/Contact Estimator ==
  q : Inport
  GRF_Estimator : MATLAB Function  TreatAsAtomicUnit=on
  Selector : Selector  InputPortWidth=4  IndexOptions=Index vector (dialog)  Indices=[2, 4]  OutputSizes=1
  Send Contact : Subsystem
  GRF : Outport
  contact : Outport  Port=2
  wires:
  GRF_Estimator/1(GRF) -> Selector/1, GRF/1
  GRF_Estimator/2(contact) -> contact/1
  q/1 -> GRF_Estimator/1(q)
  Selector/1 -> Send Contact/1(contact)

== system StateEstimation_lib/Send UDP Only/Parse Outputs ==
  outputs : Inport
  Bus Selector : BusSelector  OutputSignals=radio
  Parse_Outputs : MATLAB Function  TreatAsAtomicUnit=on
  Send IMU UDP : Subsystem
  Send JointState UDP : Subsystem
  Send Radio : Subsystem
  Send Time : Subsystem
  qwi : Outport
  wi : Outport  Port=2
  ai : Outport  Port=3
  q : Outport  Port=4
  dq : Outport  Port=5
  wires:
  Bus Selector/1 -> Send Radio/1(radio)  "<radio>"
  Parse_Outputs/5(dq) -> dq/1, Send JointState UDP/2(dq)
  outputs/1 -> Bus Selector/1, Parse_Outputs/1(outputs)
  Parse_Outputs/2(wi) -> Send IMU UDP/2(w), wi/1
  Parse_Outputs/4(q) -> q/1, Send JointState UDP/1(q)
  Parse_Outputs/1(qwi) -> qwi/1, Send IMU UDP/1(q)
  Parse_Outputs/3(ai) -> Send IMU UDP/3(a), ai/1

== system StateEstimation_lib/Send UDP Only/Send Pose UDP ==
  mu : Inport
  Sigma : Inport  Port=2
  enabled : Inport  Port=3
  "Byte Packing " : xpcutilitieslib/Byte Packing   MaskPackedDataType=uint8  MaskUnpackedDataTypes={'double'}  MaskAlignment=1
  ConstructPoseData : MATLAB Function  TreatAsAtomicUnit=on
  Digital Clock : DigitalClock  SampleTime=CassieParameters.etherCatSampleTime
  Mux1 : Mux
  Orientation EtherCAT Rate Transition10 : RateTransition  Deterministic=off  OutPortSampleTime=Pose_UDP_SampleTime
  Send : xpcrtudplib/UDP Send  ipAddressVal=Use host-target connection  localPort=-1  toAddress=10.10.10.5  toPort=25000  sampleTime=Pose_UDP_SampleTime
  Width : Width
  wires:
  Mux1/1 -> Orientation EtherCAT Rate Transition10/1
  "Byte Packing "/1 -> Width/1, Send/1
  Width/1 -> Send/2
  Orientation EtherCAT Rate Transition10/1 -> "Byte Packing "/1
  mu/1 -> Mux1/4, ConstructPoseData/1(mu)
  Sigma/1 -> ConstructPoseData/2(Sigma)
  enabled/1 -> Mux1/2
  Digital Clock/1 -> Mux1/1
  ConstructPoseData/1(pose_data) -> Mux1/3

== system StateEstimation_lib/State Estimator/Contact Estimator ==
  q : Inport
  GRF_Estimator : MATLAB Function  TreatAsAtomicUnit=on
  Selector : Selector  InputPortWidth=4  IndexOptions=Index vector (dialog)  Indices=[2, 4]  OutputSizes=1
  Send Contact : Subsystem
  GRF : Outport
  contact : Outport  Port=2
  wires:
  GRF_Estimator/1(GRF) -> Selector/1, GRF/1
  GRF_Estimator/2(contact) -> contact/1
  q/1 -> GRF_Estimator/1(q)
  Selector/1 -> Send Contact/1(contact)

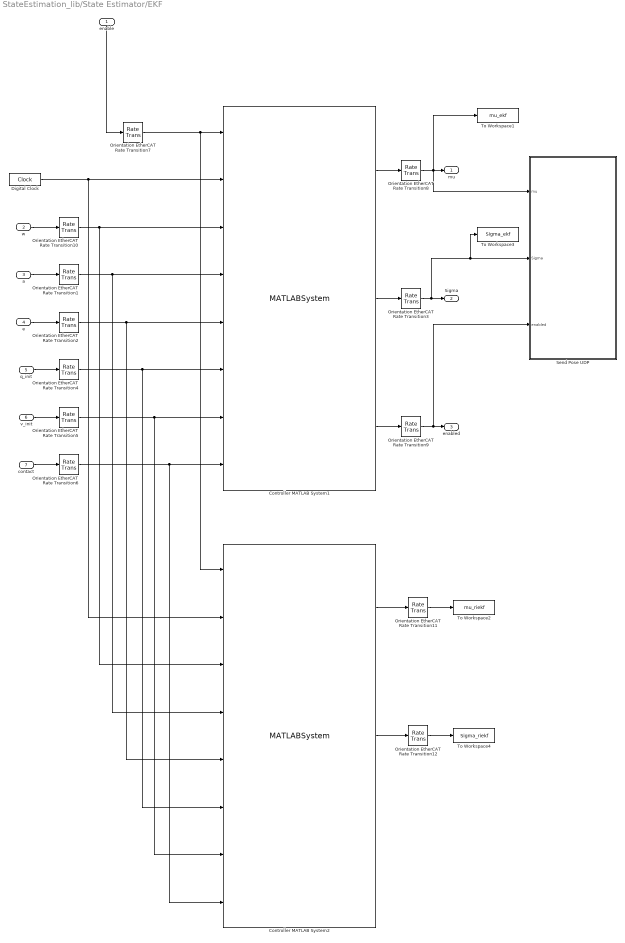
== system StateEstimation_lib/State Estimator/EKF ==
  enable : Inport
  w : Inport  Port=2
  a : Inport  Port=3
  e : Inport  Port=4
  q_init : Inport  Port=5
  v_init : Inport  Port=6
  contact : Inport  Port=7
  Controller MATLAB System1 : MATLABSystem  System=StateEstimator_EKF  static_bias_initialization=false  ekf_update_enabled=true  dt=EKF_SampleTime  enable_bias_estimation=enable_bias_estimation  gyro_noise_std=gyro_noise_std  gyro_bias_noise_std=gyro_bias_noise_std  accel_noise_std=accel_noise_std  accel_bias_noise_std=accel_bias_noise_std  contact_noise_std=contact_noise_std  encoder_noise_std=encoder_noise_std  gyro_bias_init=gyro_bias_init  accel_bias_init=accel_bias_init  SimulateUsing=Interpreted execution
      mask Type: StateEstimator_EKF
      mask Display:
      | disp('StateEstimator_EKF');
      | port_label('input',1,'EnableFilter');
      | port_label('input',2,'t');
      | port_label('input',3,'w');
      | port_label('input',4,'a');
      | port_label('input',5,'e');
      | port_label('input',6,'q_init');
      | port_label('input',7,'v_init');
      | port_label('input',8,'contact');
      | port_label('output',1,'mu');
      | port_label('output',2,'Sigma');
      | port_label('output',3,'enabled');
  Controller MATLAB System2 : MATLABSystem  System=StateEstimator_RIEKF  static_bias_initialization=false  ekf_update_enabled=true  dt=EKF_SampleTime  enable_bias_estimation=enable_bias_estimation  gyro_noise_std=gyro_noise_std  gyro_bias_noise_std=gyro_bias_noise_std  accel_noise_std=accel_noise_std  accel_bias_noise_std=accel_bias_noise_std  contact_noise_std=contact_noise_std  encoder_noise_std=encoder_noise_std  gyro_bias_init=gyro_bias_init  accel_bias_init=accel_bias_init  SimulateUsing=Interpreted execution
      mask Type: StateEstimator_RIEKF
      mask Display:
      | disp('StateEstimator_RIEKF');
      | port_label('input',1,'EnableFilter');
      | port_label('input',2,'t');
      | port_label('input',3,'w');
      | port_label('input',4,'a');
      | port_label('input',5,'e');
      | port_label('input',6,'q_init');
      | port_label('input',7,'v_init');
      | port_label('input',8,'contact');
      | port_label('output',1,'mu');
      | port_label('output',2,'Sigma');
      | port_label('output',3,'enabled');
  Digital Clock : DigitalClock  SampleTime=EKF_SampleTime
  Orientation EtherCAT Rate Transition{1..2,4..7,10} (7 alike) : RateTransition  Deterministic=off  OutPortSampleTime=EKF_SampleTime
  Orientation EtherCAT Rate Transition{3,8..9,11..12} (5 alike) : RateTransition  Deterministic=off  OutPortSampleTime=CassieParameters.etherCatSampleTime
  Send Pose UDP : Subsystem
  To Workspace1 : ToWorkspace  VariableName=mu_ekf  SaveFormat=Timeseries  SampleTime=-1
  To Workspace2 : ToWorkspace  VariableName=mu_riekf  SaveFormat=Timeseries  SampleTime=-1
  To Workspace3 : ToWorkspace  VariableName=Sigma_ekf  SaveFormat=Timeseries  SampleTime=-1
  To Workspace4 : ToWorkspace  VariableName=Sigma_riekf  SaveFormat=Timeseries  SampleTime=-1
  mu : Outport
  Sigma : Outport  Port=2
  enabled : Outport  Port=3
  wires:
  enable/1 -> Orientation EtherCAT Rate Transition7/1
  Orientation EtherCAT Rate Transition7/1 -> Controller MATLAB System2/1, Controller MATLAB System1/1
  Orientation EtherCAT Rate Transition8/1 -> To Workspace1/1, Send Pose UDP/1(mu), mu/1
  Digital Clock/1 -> Controller MATLAB System2/2, Controller MATLAB System1/2
  Orientation EtherCAT Rate Transition9/1 -> Send Pose UDP/3(enabled), enabled/1
  Controller MATLAB System1/1 -> Orientation EtherCAT Rate Transition8/1
  Controller MATLAB System1/3 -> Orientation EtherCAT Rate Transition9/1
  Orientation EtherCAT Rate Transition6/1 -> Controller MATLAB System2/8, Controller MATLAB System1/8
  Orientation EtherCAT Rate Transition5/1 -> Controller MATLAB System2/7, Controller MATLAB System1/7
  q_init/1 -> Orientation EtherCAT Rate Transition4/1
  v_init/1 -> Orientation EtherCAT Rate Transition5/1
  contact/1 -> Orientation EtherCAT Rate Transition6/1
  w/1 -> Orientation EtherCAT Rate Transition10/1
  Orientation EtherCAT Rate Transition10/1 -> Controller MATLAB System2/3, Controller MATLAB System1/3
  a/1 -> Orientation EtherCAT Rate Transition1/1
  e/1 -> Orientation EtherCAT Rate Transition2/1
  Controller MATLAB System1/2 -> Orientation EtherCAT Rate Transition3/1
  Orientation EtherCAT Rate Transition3/1 -> To Workspace3/1, Send Pose UDP/2(Sigma), Sigma/1
  Orientation EtherCAT Rate Transition1/1 -> Controller MATLAB System2/4, Controller MATLAB System1/4
  Orientation EtherCAT Rate Transition2/1 -> Controller MATLAB System2/5, Controller MATLAB System1/5
  Orientation EtherCAT Rate Transition4/1 -> Controller MATLAB System2/6, Controller MATLAB System1/6
  Controller MATLAB System2/1 -> Orientation EtherCAT Rate Transition11/1
  Orientation EtherCAT Rate Transition11/1 -> To Workspace2/1
  Controller MATLAB System2/2 -> Orientation EtherCAT Rate Transition12/1
  Orientation EtherCAT Rate Transition12/1 -> To Workspace4/1

== system StateEstimation_lib/State Estimator/Kinematic Velocity Estimator ==
  w : Inport
  q : Inport  Port=2
  dq : Inport  Port=3
  contact : Inport  Port=4
  Kinematic_Velocity : MATLAB Function  TreatAsAtomicUnit=on
  Selector2 : Selector  InputPortWidth=20  IndexOptions=Index vector (dialog)  Indices=[7:20]  OutputSizes=1
  Selector3 : Selector  InputPortWidth=20  IndexOptions=Index vector (dialog)  Indices=[7:20]  OutputSizes=1
  velocity_kinematic : Outport
  wires:
  w/1 -> Kinematic_Velocity/1(w)
  contact/1 -> Kinematic_Velocity/4(contact)
  dq/1 -> Selector3/1
  Kinematic_Velocity/1(velocity) -> velocity_kinematic/1
  q/1 -> Selector2/1
  Selector3/1 -> Kinematic_Velocity/3(e_dot)
  Selector2/1 -> Kinematic_Velocity/2(e)

== system StateEstimation_lib/State Estimator/Local Map UDP ==
  note: Local Map UDP Data Structure
      |
      | Map Information
      | double time
      | double resolution
      | double length_x
      | double length_y
      |
      | Map Center Pose
      | double position_x
      | double position_y
      | double position_z
      | double orientation_x
      | double orientation_y
      | double orientation_z
      | double orientation_w
      |
      | Update Block Data
      | double row_start_index
      | double column_start_index
      | double[100] elevation_data
  "Byte Unpacking " : xpcutilitieslib/Byte Unpacking   MaskUnpackedDataTypes={'double'}  MaskUnpackedDataSizes={[45]}  MaskAlignment=1
  Data Store Memory : DataStoreMemory  DataStoreName=local_map  ReadBeforeWriteMsg=warning  WriteAfterWriteMsg=warning  WriteAfterReadMsg=warning  ShowAdditionalParam=off
  Data Store Write : DataStoreWrite  DataStoreName=local_map
  Receive : xpcrtudplib/UDP Receive  ipAddressVal=Use host-target connection  localPort=25000  rcvWidth=45*8  rcvFmAny=off  fmAddress=10.10.10.5  sampleTime=-1
  Terminator : Terminator
  wires:
  Receive/2 -> Terminator/1
  Receive/1 -> "Byte Unpacking "/1
  "Byte Unpacking "/1 -> Data Store Write/1

== system StateEstimation_lib/State Estimator/Parse Outputs ==
  outputs : Inport
  Bus Selector : BusSelector  OutputSignals=radio
  Parse_Outputs : MATLAB Function  TreatAsAtomicUnit=on
  Send IMU UDP : Subsystem
  Send JointState UDP : Subsystem
  Send Radio : Subsystem
  Send Time : Subsystem
  qwi : Outport
  wi : Outport  Port=2
  ai : Outport  Port=3
  q : Outport  Port=4
  dq : Outport  Port=5
  wires:
  Bus Selector/1 -> Send Radio/1(radio)  "<radio>"
  Parse_Outputs/5(dq) -> dq/1, Send JointState UDP/2(dq)
  outputs/1 -> Bus Selector/1, Parse_Outputs/1(outputs)
  Parse_Outputs/2(wi) -> Send IMU UDP/2(w), wi/1
  Parse_Outputs/4(q) -> q/1, Send JointState UDP/1(q)
  Parse_Outputs/1(qwi) -> qwi/1, Send IMU UDP/1(q)
  Parse_Outputs/3(ai) -> Send IMU UDP/3(a), ai/1

== system StateEstimation_lib/State Estimator/Reconstruct State ==
  q_in : Inport
  dq_in : Inport  Port=2
  w : Inport  Port=3
  contact : Inport  Port=4
  mu_in : Inport  Port=5
  ekf_enabled : Inport  Port=6
  Construct_State : MATLAB Function  TreatAsAtomicUnit=on
  Low Pass Filter : Subsystem  TreatAsAtomicUnit=on
  Mux : Mux
  Scope 6 : slrtlib/Displays and Logging/Scope   scopeno=6  scopetype=File  autostart=on  viewmode=Numerical  formatstr='%15.6f'  grid=on  ylimits=[0,0]  nosamples=250  noprepostsamples=0  interleave=1  triggermode=FreeRun  triggersignal=1  trigsignalfromport=on  triggerlevel=0.5  triggerslope=Rising  triggerscope=1  triggersample=0  filename=ekf.dat  mode=Commit  writesize=512  autorestart=on  dynamicfilemode=off  maxwritefilesize=4000*1024^2
  q : Outport
  dq : Outport  Port=2
  velocity : Outport  Port=3
  wires:
  Low Pass Filter/1(filtered_signal) -> velocity/1
  mu_in/1 -> Construct_State/5(mu), Mux/3
  dq_in/1 -> Construct_State/2("dq ")
  Construct_State/1(q) -> q/1
  Construct_State/3(velocity) -> Mux/1, Low Pass Filter/1(signal)
  Construct_State/5(filter_selector) -> Low Pass Filter/2(selector)
  Mux/1 -> Scope 6/1
  q_in/1 -> Construct_State/1("q ")
  ekf_enabled/1 -> Construct_State/6(ekf_enabled), Mux/4
  Construct_State/2(dq) -> dq/1
  w/1 -> Construct_State/3(w)
  contact/1 -> Construct_State/4(contact)
  Construct_State/4(velocity_kinematic) -> Mux/2

== system StateEstimation_lib/State Estimator Exp Test/Contact Estimator ==
  q : Inport
  GRF_Estimator : MATLAB Function  TreatAsAtomicUnit=on
  Selector : Selector  InputPortWidth=4  IndexOptions=Index vector (dialog)  Indices=[2, 4]  OutputSizes=1
  Send Contact : Subsystem
  GRF : Outport
  contact : Outport  Port=2
  wires:
  GRF_Estimator/1(GRF) -> Selector/1, GRF/1
  GRF_Estimator/2(contact) -> contact/1
  q/1 -> GRF_Estimator/1(q)
  Selector/1 -> Send Contact/1(contact)
